simulink model "flyback"  (R2022a)
settings: Solver=VariableStepAuto  StartTime=0.0  StopTime=0.02  RelTol=1e-3
libraries: spsDiodeLib x2, spsParallelRLCBranchLib x2, spsDCVoltageSourceLib x1, spsLinearTransformerLib x1, spsMeanLib x1, spsMosfetLib x1, spsSeriesRLCBranchLib x1, spsVoltageMeasurementLib x1, spspowerguiLib x1
settings Model: Creator=kkaya674  LastModifiedBy=kkaya674

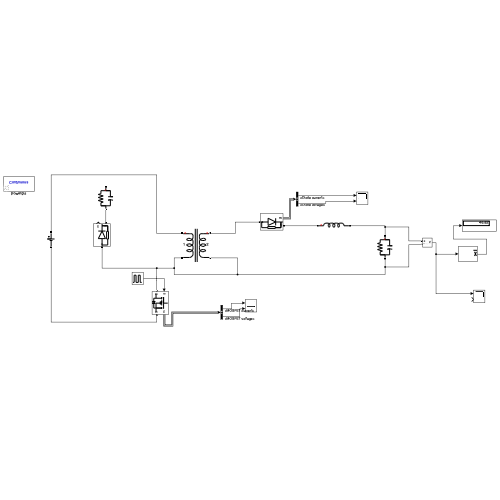
[thumbnail: Simulink's stored preview of the top-level diagram]
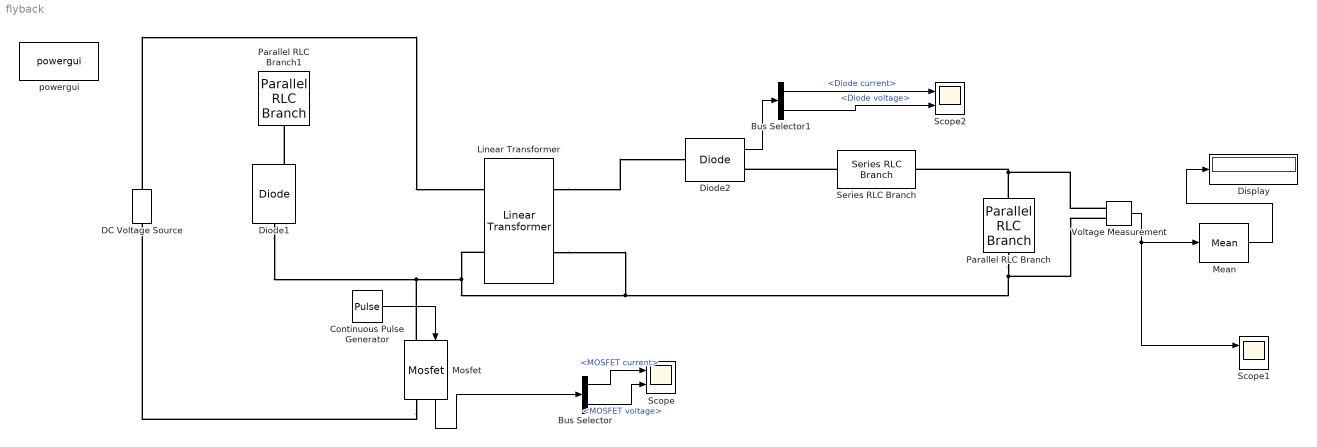
== system flyback ==
  Bus Selector : BusSelector  OutputSignals=MOSFET current,MOSFET voltage
  Bus Selector1 : BusSelector  OutputSignals=Diode current,Diode voltage
  Continuous Pulse Generator : DiscretePulseGenerator  PulseType=Time based  Period=1/10000  PulseWidth=40
  DC Voltage Source : spsDCVoltageSourceLib/DC Voltage Source  Amplitude=48  Measurements=None
  Diode1 : spsDiodeLib/Diode  Ron=0.001  Lon=0  Vf=0  IC=0  UseSnubber=0  Rs=500  Cs=250e-9  Measurements=on
  Diode2 : spsDiodeLib/Diode  Ron=0.001  Lon=0  Vf=0  IC=0  UseSnubber=0  Rs=500  Cs=250e-9  Measurements=on
  Display : Display
  Linear Transformer : spsLinearTransformerLib/Linear Transformer  UNITS=SI  NominalPower=[ 200 100e3 ]  winding1=[10 0 0]  winding2=[10 0 0]  ThreeWindings=off  winding3=[48 0 0]  RmLm=[inf 1e-4]  Measurements=Magnetization current  DataType=on
  Mean : spsMeanLib/Mean  Freq=100000  Vinit=0  Ts=0
  Mosfet : spsMosfetLib/Mosfet  Ron=0.1  Lon=0  Rd=0.01  Vfd=0  IC=0  Rs=1e5  Cs=inf  Measurements=on
  Parallel RLC Branch : spsParallelRLCBranchLib/Parallel RLC Branch  LConnTagsString=a  RConnTagsString=__new0  BranchType=RC  Resistance=5  Inductance=1e-3  SetiL0=off  InitialCurrent=0  Capacitance=100e-4  Setx0=off  InitialVoltage=0  Measurements=None
  Parallel RLC Branch1 : spsParallelRLCBranchLib/Parallel RLC Branch  LConnTagsString=a  RConnTagsString=__new0  BranchType=RC  Resistance=10  Inductance=1e-3  SetiL0=off  InitialCurrent=0  Capacitance=1e-6  Setx0=off  InitialVoltage=0  Measurements=None
  Scope : Scope  NumInputPorts=2
  Scope1 : Scope  NumInputPorts=2
  Scope2 : Scope  NumInputPorts=2
  Series RLC Branch : spsSeriesRLCBranchLib/Series RLC Branch  LConnTagsString=__new0  RConnTagsString=__new0  BranchType=L  Resistance=1  Inductance=1e-6  SetiL0=off  InitialCurrent=0  Capacitance=1e-6  Setx0=off  InitialVoltage=0  Measurements=None
  Voltage Measurement : spsVoltageMeasurementLib/Voltage Measurement  PhasorSimulation=off  OutputType=Complex  PSBequivalent=0
  powergui : spspowerguiLib/powergui  Priority=1  SimulationMode=Continuous  SampleTime=5e-5  frequency=60  Iterations=50  frequencyindice=0  Pbase=100e6  ErrMax=1e-4  UnitsV=kV  UnitsW=MW  buscounter=0  FunctionMessages=off  echomessages=off  EnableUseOfTLC=off  CurrentSourceSwitches=off  DisableSnubberDevices=off  DisableRonSwitches=off  DisableVfSwitches=off  DisplayEquations=off  AutomaticDiscreteSolvers=off  SolverType=Tustin/Backward Euler (TBE)  Interpol=off  ExternalGateDelay=off  methode=off  Ts=100  x0status=blocks  SPID=on  SwTol=0  HookPort=off  NonlinearTolerance=1e-4  nMaxIteration=100  ContinueOnMaxIteration=off  RestoreLinks=warning  ResistiveCurrentMeasurement=off  Frange=[0:2:500]  Ylog=off  Xlog=on  ShowGrid=off  save=off  variable=ZData  structure=0  ZoomFFT=off  StartTime=0.0  cycles=1  DisplayStyle=1  fundamental=60  FreqAxis=off  MaxFrequency=1000  frequencyindicesteady=1  RmsSteady=1  display=off
  wires:
  Continuous Pulse Generator/1 -> Mosfet/1
  Voltage Measurement/1 -> Mean/1, Scope1/1
  Mosfet/1 -> Bus Selector/1
  Bus Selector/1 -> Scope/1  "<MOSFET current>"
  Bus Selector/2 -> Scope/2  "<MOSFET voltage>"
  Mean/1 -> Display/1
  Diode2/1 -> Bus Selector1/1
  Bus Selector1/1 -> Scope2/1  "<Diode current>"
  Bus Selector1/2 -> Scope2/2  "<Diode voltage>"
  connections:
  Mosfet/RConn1 -- DC Voltage Source/LConn1
  DC Voltage Source/RConn1 -- Linear Transformer/LConn1
  Linear Transformer/RConn1 -- Diode2/LConn1
  Series RLC Branch/LConn1 -- Diode2/RConn1
  Voltage Measurement/LConn2 -- Mosfet/LConn1 -- Diode1/LConn1 -- Linear Transformer/LConn2 -- Linear Transformer/RConn2 -- Parallel RLC Branch/RConn1
  Parallel RLC Branch/LConn1 -- Voltage Measurement/LConn1 -- Series RLC Branch/RConn1
  Diode1/RConn1 -- Parallel RLC Branch1/RConn1
